simulink model "UpDownS_H"  (R2020a)
settings: Solver=FixedStepAuto  StartTime=0.0  StopTime=0.05  RelTol=1e-3
undefined symbols (not defined in the file): Fsw, PWMResolution
libraries: eeGeneralControl x1
settings Model: Creator=ykamatan  LastModifiedBy=ykamatan
settings SolverCC: MaxConsecutiveMinStep=10
settings DataIOCC: SaveOutput=off  SaveTime=off

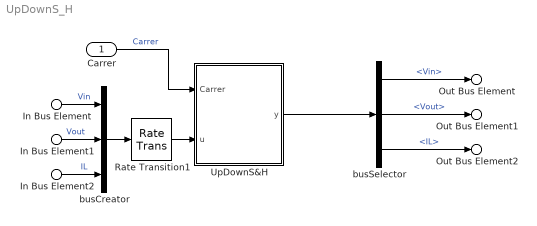
== system UpDownS_H ==
  Carrer : Inport  OutDataTypeStr=double  PortDimensions=1  SampleTime=[2e-08,0]
  In Bus Element : Inport  Port=2  PortName=Signals  Element=Vin
  In Bus Element1 : Inport  Port=2  PortName=Signals  Element=Vout
  In Bus Element2 : Inport  Port=2  PortName=Signals  Element=IL
  Rate Transition1 : RateTransition  OutPortSampleTime=1/Fsw*PWMResolution
  UpDownS&H : Subsystem  TreatAsAtomicUnit=on
  busCreator : BusCreator  Inputs=3
  busSelector : BusSelector  OutputSignals=Vin,Vout,IL
  Out Bus Element : Outport  PortName=SignalsD  Element=Vin
  Out Bus Element1 : Outport  PortName=SignalsD  Element=Vout
  Out Bus Element2 : Outport  PortName=SignalsD  Element=IL
  wires:
  busCreator/1 -> Rate Transition1/1
  In Bus Element1/1 -> busCreator/2  "Vout"
  busSelector/3 -> Out Bus Element2/1  "<IL>"
  busSelector/2 -> Out Bus Element1/1  "<Vout>"
  busSelector/1 -> Out Bus Element/1  "<Vin>"
  In Bus Element2/1 -> busCreator/3  "IL"
  In Bus Element/1 -> busCreator/1  "Vin"
  Carrer/1 -> UpDownS&H/1(Carrer)  "Carrer"
  Rate Transition1/1 -> UpDownS&H/2(u)
  UpDownS&H/1(y) -> busSelector/1

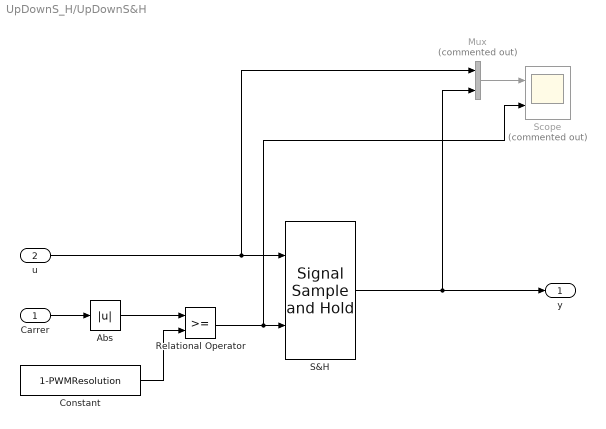
== system UpDownS_H/UpDownS&H ==
  Carrer : Inport
  u : Inport  Port=2
  Abs : Abs
  Constant : Constant  Value=1-PWMResolution
  Mux : Mux  Commented=on  Inputs=2
  Relational Operator : RelationalOperator  OutDataTypeStr=boolean  ZeroCross=off  RndMeth=Simplest
  S&H : eeGeneralControl/Signal Sample and Hold  LabelModeActiveChoice=Discrete  x0=0  Ts=-1
      settings: SourceProductBaseCode=PS
  Scope : Scope  Commented=on  NumInputPorts=2
  y : Outport
  wires:
  Constant/1 -> Relational Operator/2
  Abs/1 -> Relational Operator/1
  Mux/1 -> Scope/1
  Carrer/1 -> Abs/1
  Relational Operator/1 -> S&H/2, Scope/2
  S&H/1 -> y/1, Mux/2
  u/1 -> S&H/1, Mux/1
